simulink model "SingleJoint_Algorithm2"  (R2018b)
settings: Solver=FixedStepDiscrete  StartTime=0.0  StopTime=Inf  FixedStep=0.001  RelTol=1e-3  EnableMultiTasking=on
undefined symbols (not defined in the file): DiscIntNeverNeededParam, J3, J7, Motor_Current, Motor_Position, Motor_Velocity, Send_GUIdata
libraries: c280xlib x14, simulink x7, dspsrcs4 x1, idelinklib_common x1
(part 2 of 2)

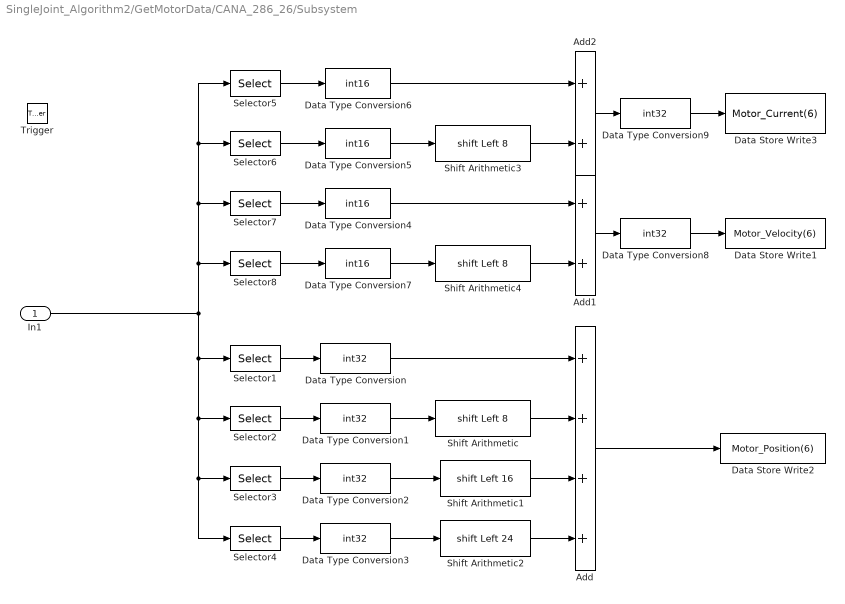
== system SingleJoint_Algorithm2/GetMotorData/CANA_286_26/Subsystem ==
  In1 : Inport
  Trigger : TriggerPort  TriggerType=function-call  VariantControl=Variant  PortDimensions=1
  Add : Sum  Inputs=4
  Add1 : Sum  Inputs=2
  Add2 : Sum  Inputs=2
  Data Store Write1 : DataStoreWrite  DataStoreName=Motor_Velocity  DataStoreElements=Motor_Velocity(6)
  Data Store Write2 : DataStoreWrite  DataStoreName=Motor_Position  DataStoreElements=Motor_Position(6)
  Data Store Write3 : DataStoreWrite  DataStoreName=Motor_Current  DataStoreElements=Motor_Current(6)
  Data Type Conversion{,1..3,8..9} (6 alike) : DataTypeConversion  OutDataTypeStr=int32
  Data Type Conversion{4..7} (4 alike) : DataTypeConversion  OutDataTypeStr=int16
  Selector1 : Selector  IndexMode=Zero-based  InputPortWidth=8  IndexOptions=Index vector (dialog)  Indices=4  OutputSizes=1
  Selector2 : Selector  IndexMode=Zero-based  InputPortWidth=8  IndexOptions=Index vector (dialog)  Indices=5  OutputSizes=1
  Selector3 : Selector  IndexMode=Zero-based  InputPortWidth=8  IndexOptions=Index vector (dialog)  Indices=6  OutputSizes=1
  Selector4 : Selector  IndexMode=Zero-based  InputPortWidth=8  IndexOptions=Index vector (dialog)  Indices=7  OutputSizes=1
  Selector5 : Selector  IndexMode=Zero-based  InputPortWidth=8  IndexOptions=Index vector (dialog)  Indices=0  OutputSizes=1
  Selector6 : Selector  IndexMode=Zero-based  InputPortWidth=8  IndexOptions=Index vector (dialog)  Indices=1  OutputSizes=1
  Selector7 : Selector  IndexMode=Zero-based  InputPortWidth=8  IndexOptions=Index vector (dialog)  Indices=2  OutputSizes=1
  Selector8 : Selector  IndexMode=Zero-based  InputPortWidth=8  IndexOptions=Index vector (dialog)  Indices=3  OutputSizes=1
  Shift Arithmetic : ArithShift  BitShiftNumber=8  BitShiftDirection=Left
  Shift Arithmetic1 : ArithShift  BitShiftNumber=16  BitShiftDirection=Left
  Shift Arithmetic2 : ArithShift  BitShiftNumber=24  BitShiftDirection=Left
  Shift Arithmetic3 : ArithShift  BitShiftNumber=8  BitShiftDirection=Left
  Shift Arithmetic4 : ArithShift  BitShiftNumber=8  BitShiftDirection=Left
  wires:
  Selector3/1 -> Data Type Conversion2/1
  Shift Arithmetic/1 -> Add/2
  Shift Arithmetic2/1 -> Add/4
  Data Type Conversion/1 -> Add/1
  Selector1/1 -> Data Type Conversion/1
  Selector4/1 -> Data Type Conversion3/1
  Add/1 -> Data Store Write2/1
  Shift Arithmetic1/1 -> Add/3
  Selector2/1 -> Data Type Conversion1/1
  Selector5/1 -> Data Type Conversion6/1
  Data Type Conversion7/1 -> Shift Arithmetic4/1
  Selector7/1 -> Data Type Conversion4/1
  Selector8/1 -> Data Type Conversion7/1
  Selector6/1 -> Data Type Conversion5/1
  In1/1 -> Selector3/1, Selector4/1, Selector2/1, Selector1/1, Selector5/1, Selector6/1, Selector7/1, Selector8/1
  Add1/1 -> Data Type Conversion8/1
  Data Type Conversion1/1 -> Shift Arithmetic/1
  Data Type Conversion2/1 -> Shift Arithmetic1/1
  Data Type Conversion3/1 -> Shift Arithmetic2/1
  Shift Arithmetic4/1 -> Add1/2
  Data Type Conversion4/1 -> Add1/1
  Data Type Conversion5/1 -> Shift Arithmetic3/1
  Data Type Conversion6/1 -> Add2/1
  Shift Arithmetic3/1 -> Add2/2
  Add2/1 -> Data Type Conversion9/1
  Data Type Conversion8/1 -> Data Store Write1/1
  Data Type Conversion9/1 -> Data Store Write3/1

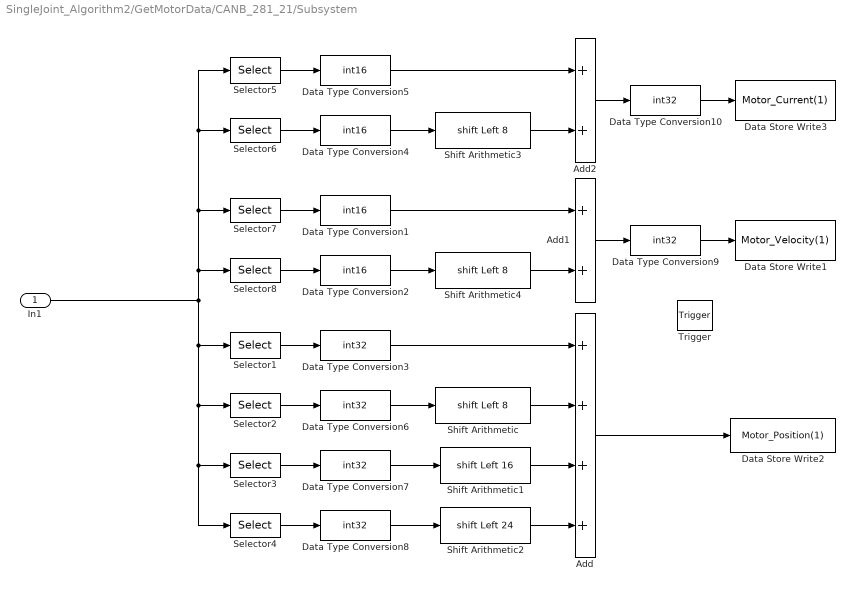
== system SingleJoint_Algorithm2/GetMotorData/CANB_281_21/Subsystem ==
  In1 : Inport
  Trigger : TriggerPort  TriggerType=function-call  VariantControl=Variant  PortDimensions=1
  Add : Sum  Inputs=4
  Add1 : Sum  Inputs=2
  Add2 : Sum  Inputs=2
  Data Store Write1 : DataStoreWrite  DataStoreName=Motor_Velocity  DataStoreElements=Motor_Velocity(1)
  Data Store Write2 : DataStoreWrite  DataStoreName=Motor_Position  DataStoreElements=Motor_Position(1)
  Data Store Write3 : DataStoreWrite  DataStoreName=Motor_Current  DataStoreElements=Motor_Current(1)
  Data Type Conversion{1..2,4..5} (4 alike) : DataTypeConversion  OutDataTypeStr=int16
  Data Type Conversion{3,6..10} (6 alike) : DataTypeConversion  OutDataTypeStr=int32
  Selector1 : Selector  IndexMode=Zero-based  InputPortWidth=8  IndexOptions=Index vector (dialog)  Indices=4  OutputSizes=1
  Selector2 : Selector  IndexMode=Zero-based  InputPortWidth=8  IndexOptions=Index vector (dialog)  Indices=5  OutputSizes=1
  Selector3 : Selector  IndexMode=Zero-based  InputPortWidth=8  IndexOptions=Index vector (dialog)  Indices=6  OutputSizes=1
  Selector4 : Selector  IndexMode=Zero-based  InputPortWidth=8  IndexOptions=Index vector (dialog)  Indices=7  OutputSizes=1
  Selector5 : Selector  IndexMode=Zero-based  InputPortWidth=8  IndexOptions=Index vector (dialog)  Indices=0  OutputSizes=1
  Selector6 : Selector  IndexMode=Zero-based  InputPortWidth=8  IndexOptions=Index vector (dialog)  Indices=1  OutputSizes=1
  Selector7 : Selector  IndexMode=Zero-based  InputPortWidth=8  IndexOptions=Index vector (dialog)  Indices=2  OutputSizes=1
  Selector8 : Selector  IndexMode=Zero-based  InputPortWidth=8  IndexOptions=Index vector (dialog)  Indices=3  OutputSizes=1
  Shift Arithmetic : ArithShift  BitShiftNumber=8  BitShiftDirection=Left
  Shift Arithmetic1 : ArithShift  BitShiftNumber=16  BitShiftDirection=Left
  Shift Arithmetic2 : ArithShift  BitShiftNumber=24  BitShiftDirection=Left
  Shift Arithmetic3 : ArithShift  BitShiftNumber=8  BitShiftDirection=Left
  Shift Arithmetic4 : ArithShift  BitShiftNumber=8  BitShiftDirection=Left
  wires:
  Data Type Conversion7/1 -> Shift Arithmetic1/1
  Shift Arithmetic/1 -> Add/2
  Selector2/1 -> Data Type Conversion6/1
  Selector3/1 -> Data Type Conversion7/1
  Shift Arithmetic2/1 -> Add/4
  Data Type Conversion3/1 -> Add/1
  Selector1/1 -> Data Type Conversion3/1
  Data Type Conversion8/1 -> Shift Arithmetic2/1
  Add/1 -> Data Store Write2/1
  Selector4/1 -> Data Type Conversion8/1
  Shift Arithmetic1/1 -> Add/3
  Data Type Conversion6/1 -> Shift Arithmetic/1
  Data Type Conversion2/1 -> Shift Arithmetic4/1
  Shift Arithmetic4/1 -> Add1/2
  Data Type Conversion1/1 -> Add1/1
  Selector7/1 -> Data Type Conversion1/1
  Selector8/1 -> Data Type Conversion2/1
  Selector6/1 -> Data Type Conversion4/1
  In1/1 -> Selector3/1, Selector4/1, Selector2/1, Selector1/1, Selector5/1, Selector6/1, Selector7/1, Selector8/1
  Add1/1 -> Data Type Conversion9/1
  Selector5/1 -> Data Type Conversion5/1
  Data Type Conversion4/1 -> Shift Arithmetic3/1
  Data Type Conversion9/1 -> Data Store Write1/1
  Shift Arithmetic3/1 -> Add2/2
  Data Type Conversion5/1 -> Add2/1
  Add2/1 -> Data Type Conversion10/1
  Data Type Conversion10/1 -> Data Store Write3/1

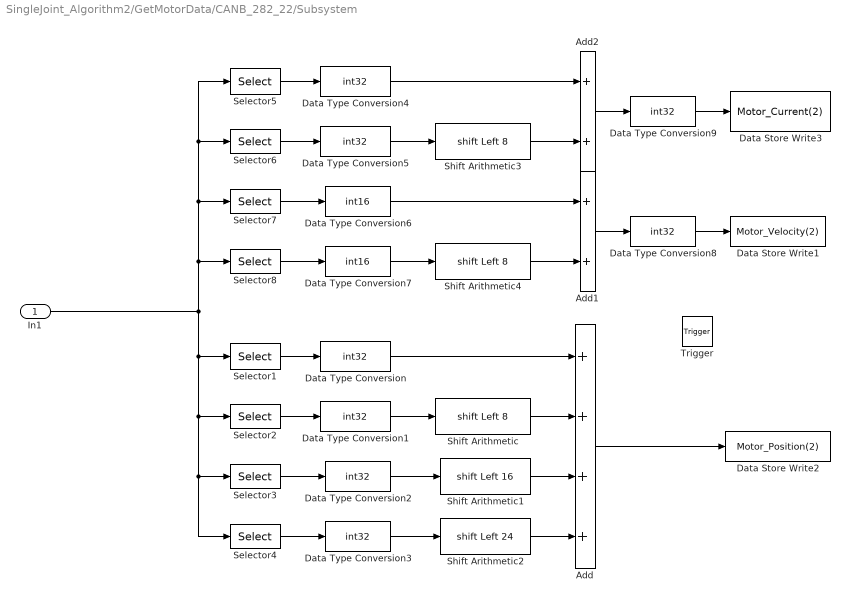
== system SingleJoint_Algorithm2/GetMotorData/CANB_282_22/Subsystem ==
  In1 : Inport
  Trigger : TriggerPort  TriggerType=function-call  VariantControl=Variant  PortDimensions=1
  Add : Sum  Inputs=4
  Add1 : Sum  Inputs=2
  Add2 : Sum  Inputs=2
  Data Store Write1 : DataStoreWrite  DataStoreName=Motor_Velocity  DataStoreElements=Motor_Velocity(2)
  Data Store Write2 : DataStoreWrite  DataStoreName=Motor_Position  DataStoreElements=Motor_Position(2)
  Data Store Write3 : DataStoreWrite  DataStoreName=Motor_Current  DataStoreElements=Motor_Current(2)
  Data Type Conversion{,1..5,8..9} (8 alike) : DataTypeConversion  OutDataTypeStr=int32
  Data Type Conversion6 : DataTypeConversion  OutDataTypeStr=int16
  Data Type Conversion7 : DataTypeConversion  OutDataTypeStr=int16
  Selector1 : Selector  IndexMode=Zero-based  InputPortWidth=8  IndexOptions=Index vector (dialog)  Indices=4  OutputSizes=1
  Selector2 : Selector  IndexMode=Zero-based  InputPortWidth=8  IndexOptions=Index vector (dialog)  Indices=5  OutputSizes=1
  Selector3 : Selector  IndexMode=Zero-based  InputPortWidth=8  IndexOptions=Index vector (dialog)  Indices=6  OutputSizes=1
  Selector4 : Selector  IndexMode=Zero-based  InputPortWidth=8  IndexOptions=Index vector (dialog)  Indices=7  OutputSizes=1
  Selector5 : Selector  IndexMode=Zero-based  InputPortWidth=8  IndexOptions=Index vector (dialog)  Indices=0  OutputSizes=1
  Selector6 : Selector  IndexMode=Zero-based  InputPortWidth=8  IndexOptions=Index vector (dialog)  Indices=1  OutputSizes=1
  Selector7 : Selector  IndexMode=Zero-based  InputPortWidth=8  IndexOptions=Index vector (dialog)  Indices=2  OutputSizes=1
  Selector8 : Selector  IndexMode=Zero-based  InputPortWidth=8  IndexOptions=Index vector (dialog)  Indices=3  OutputSizes=1
  Shift Arithmetic : ArithShift  BitShiftNumber=8  BitShiftDirection=Left
  Shift Arithmetic1 : ArithShift  BitShiftNumber=16  BitShiftDirection=Left
  Shift Arithmetic2 : ArithShift  BitShiftNumber=24  BitShiftDirection=Left
  Shift Arithmetic3 : ArithShift  BitShiftNumber=8  BitShiftDirection=Left
  Shift Arithmetic4 : ArithShift  BitShiftNumber=8  BitShiftDirection=Left
  wires:
  Data Type Conversion2/1 -> Shift Arithmetic1/1
  Shift Arithmetic/1 -> Add/2
  Selector2/1 -> Data Type Conversion1/1
  Selector3/1 -> Data Type Conversion2/1
  Shift Arithmetic2/1 -> Add/4
  Data Type Conversion/1 -> Add/1
  Selector1/1 -> Data Type Conversion/1
  Data Type Conversion3/1 -> Shift Arithmetic2/1
  Add/1 -> Data Store Write2/1
  Selector4/1 -> Data Type Conversion3/1
  Shift Arithmetic1/1 -> Add/3
  Data Type Conversion1/1 -> Shift Arithmetic/1
  In1/1 -> Selector3/1, Selector4/1, Selector2/1, Selector1/1, Selector8/1, Selector7/1, Selector6/1, Selector5/1
  Shift Arithmetic4/1 -> Add1/2
  Add1/1 -> Data Type Conversion8/1
  Data Type Conversion5/1 -> Shift Arithmetic3/1
  Selector8/1 -> Data Type Conversion7/1
  Data Type Conversion6/1 -> Add1/1
  Selector6/1 -> Data Type Conversion5/1
  Data Type Conversion7/1 -> Shift Arithmetic4/1
  Selector5/1 -> Data Type Conversion4/1
  Selector7/1 -> Data Type Conversion6/1
  Data Type Conversion8/1 -> Data Store Write1/1
  Shift Arithmetic3/1 -> Add2/2
  Data Type Conversion4/1 -> Add2/1
  Add2/1 -> Data Type Conversion9/1
  Data Type Conversion9/1 -> Data Store Write3/1

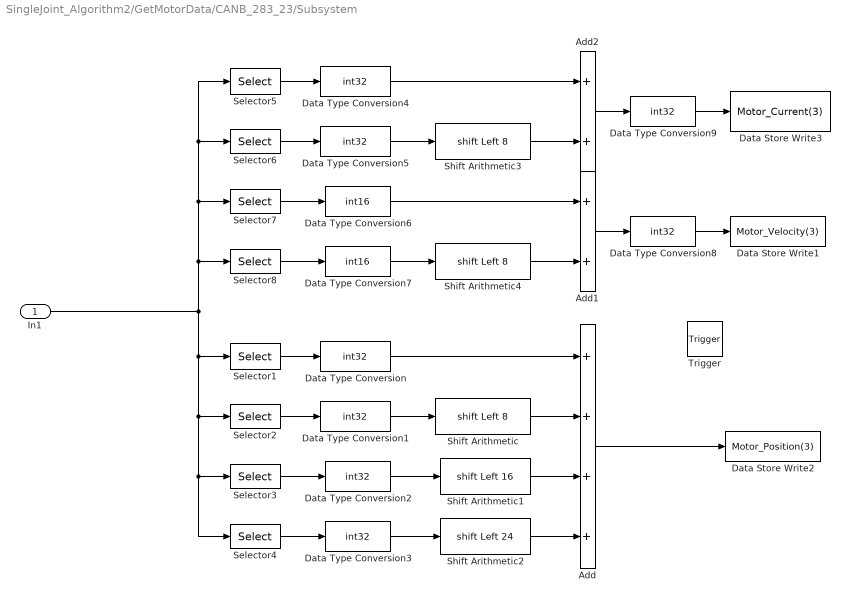
== system SingleJoint_Algorithm2/GetMotorData/CANB_283_23/Subsystem ==
  In1 : Inport
  Trigger : TriggerPort  TriggerType=function-call  VariantControl=Variant  PortDimensions=1
  Add : Sum  Inputs=4
  Add1 : Sum  Inputs=2
  Add2 : Sum  Inputs=2
  Data Store Write1 : DataStoreWrite  DataStoreName=Motor_Velocity  DataStoreElements=Motor_Velocity(3)
  Data Store Write2 : DataStoreWrite  DataStoreName=Motor_Position  DataStoreElements=Motor_Position(3)
  Data Store Write3 : DataStoreWrite  DataStoreName=Motor_Current  DataStoreElements=Motor_Current(3)
  Data Type Conversion{,1..5,8..9} (8 alike) : DataTypeConversion  OutDataTypeStr=int32
  Data Type Conversion6 : DataTypeConversion  OutDataTypeStr=int16
  Data Type Conversion7 : DataTypeConversion  OutDataTypeStr=int16
  Selector1 : Selector  IndexMode=Zero-based  InputPortWidth=8  IndexOptions=Index vector (dialog)  Indices=4  OutputSizes=1
  Selector2 : Selector  IndexMode=Zero-based  InputPortWidth=8  IndexOptions=Index vector (dialog)  Indices=5  OutputSizes=1
  Selector3 : Selector  IndexMode=Zero-based  InputPortWidth=8  IndexOptions=Index vector (dialog)  Indices=6  OutputSizes=1
  Selector4 : Selector  IndexMode=Zero-based  InputPortWidth=8  IndexOptions=Index vector (dialog)  Indices=7  OutputSizes=1
  Selector5 : Selector  IndexMode=Zero-based  InputPortWidth=8  IndexOptions=Index vector (dialog)  Indices=0  OutputSizes=1
  Selector6 : Selector  IndexMode=Zero-based  InputPortWidth=8  IndexOptions=Index vector (dialog)  Indices=1  OutputSizes=1
  Selector7 : Selector  IndexMode=Zero-based  InputPortWidth=8  IndexOptions=Index vector (dialog)  Indices=2  OutputSizes=1
  Selector8 : Selector  IndexMode=Zero-based  InputPortWidth=8  IndexOptions=Index vector (dialog)  Indices=3  OutputSizes=1
  Shift Arithmetic : ArithShift  BitShiftNumber=8  BitShiftDirection=Left
  Shift Arithmetic1 : ArithShift  BitShiftNumber=16  BitShiftDirection=Left
  Shift Arithmetic2 : ArithShift  BitShiftNumber=24  BitShiftDirection=Left
  Shift Arithmetic3 : ArithShift  BitShiftNumber=8  BitShiftDirection=Left
  Shift Arithmetic4 : ArithShift  BitShiftNumber=8  BitShiftDirection=Left
  wires:
  Data Type Conversion2/1 -> Shift Arithmetic1/1
  Shift Arithmetic/1 -> Add/2
  Selector2/1 -> Data Type Conversion1/1
  Selector3/1 -> Data Type Conversion2/1
  Shift Arithmetic2/1 -> Add/4
  Data Type Conversion/1 -> Add/1
  Selector1/1 -> Data Type Conversion/1
  Data Type Conversion3/1 -> Shift Arithmetic2/1
  Add/1 -> Data Store Write2/1
  Selector4/1 -> Data Type Conversion3/1
  Shift Arithmetic1/1 -> Add/3
  Data Type Conversion1/1 -> Shift Arithmetic/1
  Selector6/1 -> Data Type Conversion5/1
  Selector5/1 -> Data Type Conversion4/1
  Data Type Conversion7/1 -> Shift Arithmetic4/1
  Data Type Conversion6/1 -> Add1/1
  Selector7/1 -> Data Type Conversion6/1
  Selector8/1 -> Data Type Conversion7/1
  Data Type Conversion5/1 -> Shift Arithmetic3/1
  In1/1 -> Selector3/1, Selector4/1, Selector2/1, Selector1/1, Selector5/1, Selector6/1, Selector7/1, Selector8/1
  Add1/1 -> Data Type Conversion8/1
  Shift Arithmetic4/1 -> Add1/2
  Data Type Conversion8/1 -> Data Store Write1/1
  Shift Arithmetic3/1 -> Add2/2
  Data Type Conversion4/1 -> Add2/1
  Add2/1 -> Data Type Conversion9/1
  Data Type Conversion9/1 -> Data Store Write3/1

== system SingleJoint_Algorithm2/接收上位机的数据/Subsystem/Joint1 ==
  Joint1 : Inport
  Action Port : ActionPort  ActionType=case
  Data Store Write2 : DataStoreWrite  DataStoreName=J1
  wires:
  Joint1/1 -> Data Store Write2/1

== system SingleJoint_Algorithm2/接收上位机的数据/Subsystem/Joint2 ==
  Joint2 : Inport
  Action Port : ActionPort  ActionType=case
  Data Store Write2 : DataStoreWrite  DataStoreName=J2
  wires:
  Joint2/1 -> Data Store Write2/1

== system SingleJoint_Algorithm2/接收上位机的数据/Subsystem/Joint3 ==
  Joint3 : Inport
  Action Port : ActionPort  ActionType=case
  Data Store Write2 : DataStoreWrite  DataStoreName=J3
  wires:
  Joint3/1 -> Data Store Write2/1

== system SingleJoint_Algorithm2/接收上位机的数据/Subsystem/Joint4 ==
  Joint4 : Inport
  Action Port : ActionPort  ActionType=case
  Data Store Write2 : DataStoreWrite  DataStoreName=J4
  wires:
  Joint4/1 -> Data Store Write2/1

== system SingleJoint_Algorithm2/接收上位机的数据/Subsystem/Joint5 ==
  Joint5 : Inport
  Action Port : ActionPort  ActionType=case
  Data Store Write2 : DataStoreWrite  DataStoreName=J5
  wires:
  Joint5/1 -> Data Store Write2/1

== system SingleJoint_Algorithm2/接收上位机的数据/Subsystem/Joint6 ==
  Joint6 : Inport
  Action Port : ActionPort  ActionType=case
  Data Store Write2 : DataStoreWrite  DataStoreName=J6
  wires:
  Joint6/1 -> Data Store Write2/1

== system SingleJoint_Algorithm2/接收上位机的数据/Subsystem/Joint7 ==
  Joint7 : Inport
  Action Port : ActionPort  ActionType=case
  Data Store Write2 : DataStoreWrite  DataStoreName=J7
  wires:
  Joint7/1 -> Data Store Write2/1

== system SingleJoint_Algorithm2/接收上位机的数据/获取用户命令/消息校验 ==
  数据 : Inport
  Add : Sum  Inputs=8
  Constant : Constant  Value=[0 0 0 0 0 0 0 0 0]  OutDataTypeStr=uint16
  Data Type Conversion : DataTypeConversion  OutDataTypeStr=uint16
  Demux : Demux  Outputs=9
  Relational Operator : RelationalOperator  Operator===  OutDataTypeStr=boolean  RndMeth=Simplest
  Switch : Switch  Criteria=u2 > Threshold
  消息 : Outport
  使能 : Outport  Port=2
  wires:
  数据/1 -> Switch/1, Demux/1
  Demux/1 -> Add/1
  Demux/2 -> Add/2
  Demux/3 -> Add/3
  Demux/4 -> Add/4
  Demux/5 -> Add/5
  Demux/6 -> Add/6
  Demux/7 -> Add/7
  Demux/8 -> Add/8
  Add/1 -> Data Type Conversion/1
  Data Type Conversion/1 -> Relational Operator/1
  Demux/9 -> Relational Operator/2
  Switch/1 -> 消息/1
  Constant/1 -> Switch/3
  Relational Operator/1 -> Switch/2, 使能/1

== system SingleJoint_Algorithm2/AdaptionController/AdapitionController/Controller/SolveTau ==
  note: $\dot\hat\omega=-\lambda f^Ts$
  note: $f\hat\omega$
  note: $K_Ds$
  note: $\Gamma_0\eta_1$
  Gamma0 eta1 : Inport
  f : Inport  Port=2
  lambda : Inport  Port=3
  KD : Inport  Port=4
  s : Inport  Port=5
  6 : Gain  Gain=-1  OutDataTypeStr=double
  Add : Sum  Inputs=++-
  Discrete-Time Integrator2 : DiscreteIntegrator  SampleTime=-1  LimitOutput=on  UpperSaturationLimit=[1000;1000;1000;1000;1000;1000;1000;]  LowerSaturationLimit=[-1000;-1000;-1000;-1000;-1000;-1000;-1000;]  ICPrevOutput=DiscIntNeverNeededParam  ICPrevScaledInput=DiscIntNeverNeededParam
  Math Function2 : Math  Operator=transpose  SaturateOnIntegerOverflow=on
  Product5 : Product
  Product6 : Product  Inputs=3
  Product7 : Product  Multiplication=Matrix(*)
  transpose : Reshape  OutputDimensionality=Customize  OutputDimensions=[1,7]
  Tau : Outport
  wires:
  f/1 -> Math Function2/1, transpose/1
  Product6/1 -> Discrete-Time Integrator2/1
  Product7/1 -> Add/2
  Product5/1 -> Add/3
  lambda/1 -> 6/1
  Math Function2/1 -> Product6/1
  Discrete-Time Integrator2/1 -> Product7/2
  6/1 -> Product6/2
  s/1 -> Product6/3, Product5/1
  transpose/1 -> Product7/1
  KD/1 -> Product5/2
  Gamma0 eta1/1 -> Add/1
  Add/1 -> Tau/1

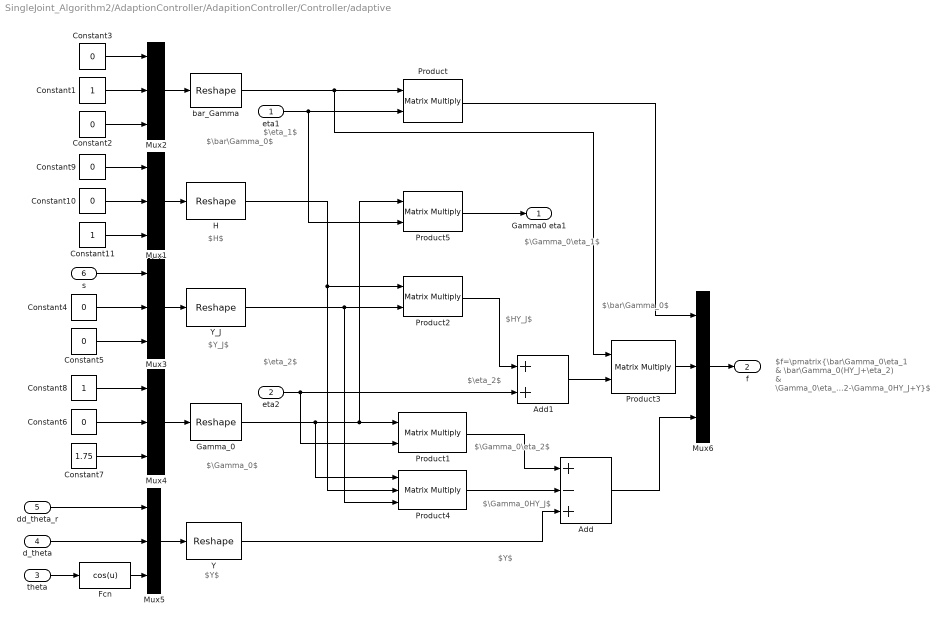
== system SingleJoint_Algorithm2/AdaptionController/AdapitionController/Controller/adaptive ==
  note: $\eta_2$
  note: $\bar\Gamma_0$
  note: $\Gamma_0$
  note: $\eta_1$
  note: $\Gamma_0\eta_1$
  note: $H$
  note: $Y_J$
  note: $Y$
  note: $HY_J$
  note: $\Gamma_0\eta_2$
  note: $\Gamma_0HY_J$
  note: $Y$
  note: $\eta_2$
  note: $\bar\Gamma_0$
  note: $f=\pmatrix{\bar\Gamma_0\eta_1 & \bar\Gamma_0(HY_J+\eta_2) & \Gamma_0\eta_2-\Gamma_0HY_J+Y}$
  eta1 : Inport
  eta2 : Inport  Port=2
  theta : Inport  Port=3
  d_theta : Inport  Port=4
  dd_theta_r : Inport  Port=5
  s : Inport  Port=6
  Add : Sum  Inputs=+-+
  Add1 : Sum
  Constant1 : Constant
  Constant{2..6,9..10} (7 alike) : Constant  Value=0
  Constant11 : Constant
  Constant7 : Constant  Value=1.75
  Constant8 : Constant
  Fcn : Fcn  Expr=cos(u)
  Gamma_0 : Reshape  OutputDimensionality=Customize  OutputDimensions=[1,3]
  H : Reshape  OutputDimensionality=Customize  OutputDimensions=[3,1]
  Mux{1..6} (6 alike) : Mux  Inputs=3
  Product{,1..3,5} (5 alike) : Product  Multiplication=Matrix(*)
  Product4 : Product  Inputs=3  Multiplication=Matrix(*)
  Y : Reshape  OutputDimensionality=Customize  OutputDimensions=[1,3]
  Y_J : Reshape  OutputDimensionality=Customize  OutputDimensions=[1,3]
  bar_Gamma : Reshape  OutputDimensionality=Customize  OutputDimensions=[1,3]
  Gamma0 eta1 : Outport
  f : Outport  Port=2
  wires:
  H/1 -> Product4/2, Product2/1
  Mux1/1 -> H/1
  Constant11/1 -> Mux1/3
  Constant10/1 -> Mux1/2
  Constant9/1 -> Mux1/1
  bar_Gamma/1 -> Product/1, Product3/1
  Constant2/1 -> Mux2/3
  Constant1/1 -> Mux2/2
  Constant3/1 -> Mux2/1
  Mux2/1 -> bar_Gamma/1
  eta1/1 -> Product5/2, Product/2
  Mux3/1 -> Y_J/1
  Constant5/1 -> Mux3/3
  Constant4/1 -> Mux3/2
  s/1 -> Mux3/1
  Y_J/1 -> Product2/2, Product4/3
  Product2/1 -> Add1/1
  eta2/1 -> Product1/2, Add1/2
  Add1/1 -> Product3/2
  Mux4/1 -> Gamma_0/1
  Constant7/1 -> Mux4/3
  Constant6/1 -> Mux4/2
  Constant8/1 -> Mux4/1
  Gamma_0/1 -> Product4/1, Product5/1, Product1/1
  dd_theta_r/1 -> Mux5/1
  d_theta/1 -> Mux5/2
  theta/1 -> Fcn/1
  Fcn/1 -> Mux5/3
  Mux5/1 -> Y/1
  Y/1 -> Add/3
  Product4/1 -> Add/2
  Product1/1 -> Add/1
  Product3/1 -> Mux6/2
  Product/1 -> Mux6/1
  Mux6/1 -> f/1
  Add/1 -> Mux6/3
  Product5/1 -> Gamma0 eta1/1

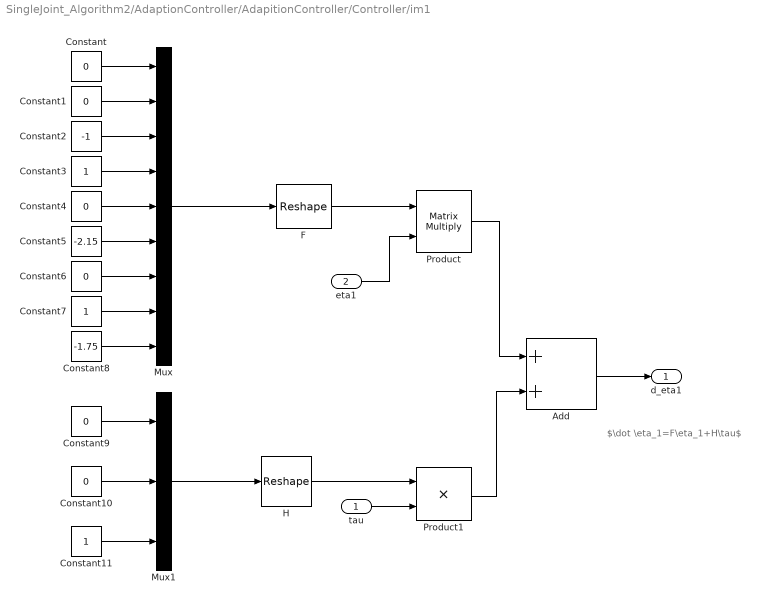
== system SingleJoint_Algorithm2/AdaptionController/AdapitionController/Controller/im1 ==
  note: $\dot \eta_1=F\eta_1+H\tau$
  tau : Inport
  eta1 : Inport  Port=2
  Add : Sum
  Constant{,1,4,6,9..10} (6 alike) : Constant  Value=0
  Constant11 : Constant
  Constant2 : Constant  Value=-1
  Constant3 : Constant
  Constant5 : Constant  Value=-2.15
  Constant7 : Constant
  Constant8 : Constant  Value=-1.75
  F : Reshape  OutputDimensionality=Customize  OutputDimensions=[3,3]
  H : Reshape  OutputDimensionality=Customize  OutputDimensions=[3,1]
  Mux : Mux  Inputs=9
  Mux1 : Mux  Inputs=3
  Product : Product  Multiplication=Matrix(*)
  Product1 : Product
  d_eta1 : Outport
  wires:
  Constant/1 -> Mux/1
  Constant1/1 -> Mux/2
  Constant2/1 -> Mux/3
  Constant3/1 -> Mux/4
  Constant4/1 -> Mux/5
  Constant5/1 -> Mux/6
  Constant6/1 -> Mux/7
  Constant7/1 -> Mux/8
  Constant8/1 -> Mux/9
  Mux/1 -> F/1
  F/1 -> Product/1
  Product/1 -> Add/1
  Constant9/1 -> Mux1/1
  Constant10/1 -> Mux1/2
  Constant11/1 -> Mux1/3
  Mux1/1 -> H/1
  H/1 -> Product1/1
  tau/1 -> Product1/2
  Product1/1 -> Add/2
  Add/1 -> d_eta1/1
  eta1/1 -> Product/2

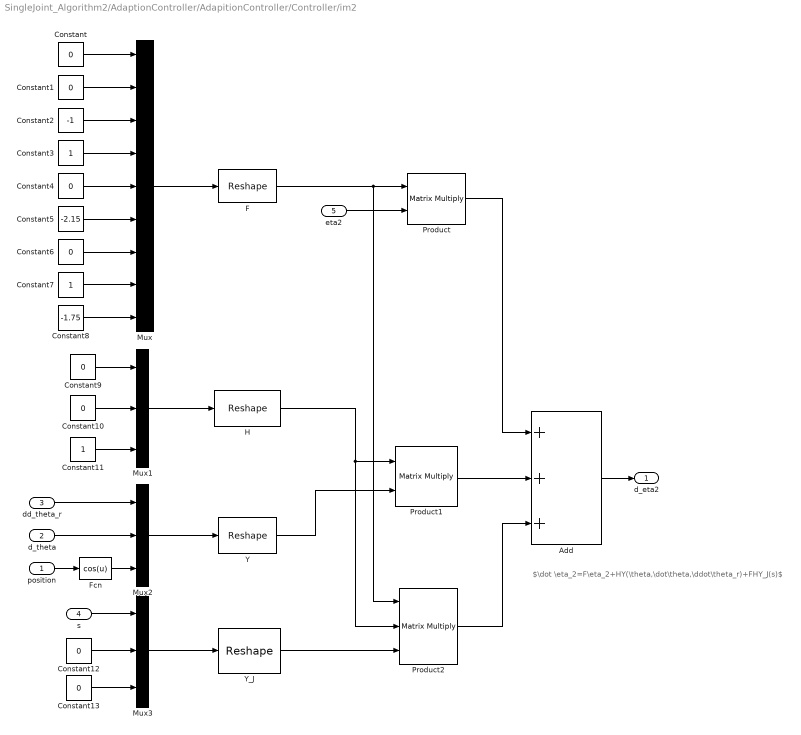
== system SingleJoint_Algorithm2/AdaptionController/AdapitionController/Controller/im2 ==
  note: $\dot \eta_2=F\eta_2+HY(\theta,\dot\theta,\ddot\theta_r)+FHY_J(s)$
  position : Inport
  d_theta : Inport  Port=2
  dd_theta_r : Inport  Port=3
  s : Inport  Port=4
  eta2 : Inport  Port=5
  Add : Sum  Inputs=+++
  Constant{,1,4,6,9..10,12..13} (8 alike) : Constant  Value=0
  Constant11 : Constant
  Constant2 : Constant  Value=-1
  Constant3 : Constant
  Constant5 : Constant  Value=-2.15
  Constant7 : Constant
  Constant8 : Constant  Value=-1.75
  F : Reshape  OutputDimensionality=Customize  OutputDimensions=[3,3]
  Fcn : Fcn  Expr=cos(u)
  H : Reshape  OutputDimensionality=Customize  OutputDimensions=[3,1]
  Mux : Mux  Inputs=9
  Mux1 : Mux  Inputs=3
  Mux2 : Mux  Inputs=3
  Mux3 : Mux  Inputs=3
  Product : Product  Multiplication=Matrix(*)
  Product1 : Product  Multiplication=Matrix(*)
  Product2 : Product  Inputs=3  Multiplication=Matrix(*)
  Y : Reshape  OutputDimensionality=Customize  OutputDimensions=[1,3]
  Y_J : Reshape  OutputDimensionality=Customize  OutputDimensions=[1,3]
  d_eta2 : Outport
  wires:
  eta2/1 -> Product/2
  Add/1 -> d_eta2/1
  Product1/1 -> Add/2
  H/1 -> Product2/2, Product1/1
  Mux1/1 -> H/1
  Constant11/1 -> Mux1/3
  Constant10/1 -> Mux1/2
  Constant9/1 -> Mux1/1
  Product/1 -> Add/1
  F/1 -> Product2/1, Product/1
  Mux/1 -> F/1
  Constant8/1 -> Mux/9
  Constant7/1 -> Mux/8
  Constant6/1 -> Mux/7
  Constant5/1 -> Mux/6
  Constant4/1 -> Mux/5
  Constant3/1 -> Mux/4
  Constant2/1 -> Mux/3
  Constant1/1 -> Mux/2
  Constant/1 -> Mux/1
  dd_theta_r/1 -> Mux2/1
  d_theta/1 -> Mux2/2
  position/1 -> Fcn/1
  Fcn/1 -> Mux2/3
  Mux2/1 -> Y/1
  Y/1 -> Product1/2
  s/1 -> Mux3/1
  Constant12/1 -> Mux3/2
  Constant13/1 -> Mux3/3
  Mux3/1 -> Y_J/1
  Y_J/1 -> Product2/3
  Product2/1 -> Add/3

== system SingleJoint_Algorithm2/AdaptionController/AdapitionController/Error/Subsystem ==
  note: $e_1(t)=\theta(t)-\theta_d(t)$
  q1 : Inport
  gian : Inport  Port=2
  Enable : EnablePort
  Product : Product
  Sum5 : Sum  Inputs=+-|
  ref_signal : dspsrcs4/Sine Wave  Amplitude=1  Frequency=Freq  Phase=0  SampleMode=Discrete  OutComplex=Real  CompMethod=Trigonometric fcn  TableSize=Speed  SampleTime=SimpleTime  SamplesPerFrame=1  ResetState=Restart at time zero  OutputFrames=on  dataType=double  wordLen=16  udDataType=sfix(16)  fracBitsMode=Best precision  numFracBits=15  OutDataTypeStr=double  LastOutDataTypeStr=double
  e1 : Outport
  qd : Outport  Port=2
  wires:
  ref_signal/1 -> Product/1
  Product/1 -> Sum5/2, qd/1
  gian/1 -> Product/2
  q1/1 -> Sum5/1
  Sum5/1 -> e1/1

== system SingleJoint_Algorithm2/AdaptionController/DriverOneMotor/BottomDriver/Joint1 ==
  In6 : Inport
  Action Port : ActionPort
  Constant : Constant  Value=0  OutDataTypeStr=uint8
  Data Store Write : DataStoreWrite  DataStoreName=One_TXD
  eCANB_301_7 : c280xlib/eCAN Transmit  chipFamily=C280x  useModule=eCAN_B  mailboxNo=7  messageID=hex2dec('301')  messageType=Standard (11-bit identifier)  enableBlockingMode=off  postInterrupt=off  interruptLine=0
      settings: SourceProductName=Embedded Coder Support Package for Texas Instruments C2000 Processors  SourceProductBaseCode=TIC2000
  wires:
  In6/1 -> eCANB_301_7/1
  Constant/1 -> Data Store Write/1

== system SingleJoint_Algorithm2/AdaptionController/DriverOneMotor/BottomDriver/Joint2 ==
  In1 : Inport
  Action Port : ActionPort
  Constant : Constant  Value=0  OutDataTypeStr=uint8
  Data Store Write : DataStoreWrite  DataStoreName=One_TXD
  eCANB _302_7 : c280xlib/eCAN Transmit  chipFamily=C280x  useModule=eCAN_B  mailboxNo=7  messageID=hex2dec('302')  messageType=Standard (11-bit identifier)  enableBlockingMode=off  postInterrupt=off  interruptLine=0
      settings: SourceProductName=Embedded Coder Support Package for Texas Instruments C2000 Processors  SourceProductBaseCode=TIC2000
  wires:
  In1/1 -> eCANB _302_7/1
  Constant/1 -> Data Store Write/1

== system SingleJoint_Algorithm2/AdaptionController/DriverOneMotor/BottomDriver/Joint3 ==
  In1 : Inport
  Action Port : ActionPort  ActionType=case
  Constant : Constant  Value=0  OutDataTypeStr=uint8
  Data Store Write : DataStoreWrite  DataStoreName=One_TXD
  eCANB _303_7 : c280xlib/eCAN Transmit  chipFamily=C280x  useModule=eCAN_B  mailboxNo=7  messageID=hex2dec('303')  messageType=Standard (11-bit identifier)  enableBlockingMode=off  postInterrupt=off  interruptLine=0
      settings: SourceProductName=Embedded Coder Support Package for Texas Instruments C2000 Processors  SourceProductBaseCode=TIC2000
  wires:
  In1/1 -> eCANB _303_7/1
  Constant/1 -> Data Store Write/1

== system SingleJoint_Algorithm2/AdaptionController/DriverOneMotor/BottomDriver/Joint4 ==
  In1 : Inport
  Action Port : ActionPort
  Constant : Constant  Value=0  OutDataTypeStr=uint8
  Data Store Write : DataStoreWrite  DataStoreName=One_TXD
  eCANA_304_7 : c280xlib/eCAN Transmit  chipFamily=C280x  useModule=eCAN_A  mailboxNo=7  messageID=hex2dec('304')  messageType=Standard (11-bit identifier)  enableBlockingMode=off  postInterrupt=off  interruptLine=0
      settings: SourceProductName=Embedded Coder Support Package for Texas Instruments C2000 Processors  SourceProductBaseCode=TIC2000
  wires:
  In1/1 -> eCANA_304_7/1
  Constant/1 -> Data Store Write/1

== system SingleJoint_Algorithm2/AdaptionController/DriverOneMotor/BottomDriver/Joint5 ==
  In1 : Inport
  Action Port : ActionPort
  Constant : Constant  Value=0  OutDataTypeStr=uint8
  Data Store Write : DataStoreWrite  DataStoreName=One_TXD
  eCANA_305_7 : c280xlib/eCAN Transmit  chipFamily=C280x  useModule=eCAN_A  mailboxNo=7  messageID=hex2dec('305')  messageType=Standard (11-bit identifier)  enableBlockingMode=off  postInterrupt=off  interruptLine=0
      settings: SourceProductName=Embedded Coder Support Package for Texas Instruments C2000 Processors  SourceProductBaseCode=TIC2000
  wires:
  In1/1 -> eCANA_305_7/1
  Constant/1 -> Data Store Write/1

== system SingleJoint_Algorithm2/AdaptionController/DriverOneMotor/BottomDriver/Joint6 ==
  In1 : Inport
  Action Port : ActionPort
  Constant : Constant  Value=0  OutDataTypeStr=uint8
  Data Store Write : DataStoreWrite  DataStoreName=One_TXD
  eCANA_306_7 : c280xlib/eCAN Transmit  chipFamily=C280x  useModule=eCAN_A  mailboxNo=7  messageID=hex2dec('306')  messageType=Standard (11-bit identifier)  enableBlockingMode=off  postInterrupt=off  interruptLine=0
      settings: SourceProductName=Embedded Coder Support Package for Texas Instruments C2000 Processors  SourceProductBaseCode=TIC2000
  wires:
  In1/1 -> eCANA_306_7/1
  Constant/1 -> Data Store Write/1

== system SingleJoint_Algorithm2/AdaptionController/DriverOneMotor/驱动器指令/DriveOder/BG ==
  note: 命令
  note: 电流
  note: 位
      | 置
  f : TriggerPort  TriggerType=function-call  VariantControl=(inherit)
      settings: CopyFcn=Stateflow.SLINSF.SimulinkMan.removeBlockPreDeleteFcn  PreDeleteFcn=Stateflow.SLINSF.SimulinkMan.unsafePredeleteFcn
  Constant1 : Constant  Value=hex2dec('47')  OutDataTypeStr=uint8
  Constant2 : Constant  Value=0  VectorParams1D=off  OutDataTypeStr=uint8  SampleTime=-1
  Constant3 : Constant  Value=0  VectorParams1D=off  OutDataTypeStr=uint8  SampleTime=-1
  Constant6 : Constant  OutDataTypeStr=uint8
  Constant8 : Constant  Value=hex2dec('42')  OutDataTypeStr=uint8
  Data Store Write : DataStoreWrite  DataStoreName=One_TXD
  Data Type Conversion : DataTypeConversion  OutDataTypeStr=uint16
  Data Type Conversion{1..6} (6 alike) : DataTypeConversion  OutDataTypeStr=uint8
  Mux3 : Mux  Inputs=8
  Shift Arithmetic1 : ArithShift  BitShiftNumber=8  BitShiftDirection=Right
  Shift Arithmetic2 : ArithShift  BitShiftNumber=16  BitShiftDirection=Right
  Shift Arithmetic3 : ArithShift  BitShiftNumber=24  BitShiftDirection=Right
  Shift Arithmetic4 : ArithShift  BitShiftNumber=8  BitShiftDirection=Right
  MSG : Outport  OutDataTypeStr=uint16  PortDimensions=8
  wires:
  Constant6/1 -> Data Store Write/1
  Data Type Conversion2/1 -> Mux3/5
  Constant3/1 -> Data Type Conversion2/1, Shift Arithmetic1/1, Shift Arithmetic2/1, Shift Arithmetic3/1
  Data Type Conversion5/1 -> Mux3/8
  Data Type Conversion4/1 -> Mux3/7
  Constant1/1 -> Mux3/2
  Constant8/1 -> Mux3/1
  Mux3/1 -> Data Type Conversion/1
  Data Type Conversion6/1 -> Mux3/4
  Data Type Conversion3/1 -> Mux3/6
  Shift Arithmetic2/1 -> Data Type Conversion4/1
  Data Type Conversion1/1 -> Mux3/3
  Constant2/1 -> Shift Arithmetic4/1, Data Type Conversion1/1
  Shift Arithmetic3/1 -> Data Type Conversion5/1
  Shift Arithmetic4/1 -> Data Type Conversion6/1
  Shift Arithmetic1/1 -> Data Type Conversion3/1
  Data Type Conversion/1 -> MSG/1

== system SingleJoint_Algorithm2/AdaptionController/DriverOneMotor/驱动器指令/DriveOder/TF ==
  note: 命令
  note: 位
      | 置
  note: 电流
  Current : Inport  OutDataTypeStr=uint16  PortDimensions=1
  f : TriggerPort  TriggerType=function-call  VariantControl=(inherit)
      settings: CopyFcn=Stateflow.SLINSF.SimulinkMan.removeBlockPreDeleteFcn  PreDeleteFcn=Stateflow.SLINSF.SimulinkMan.unsafePredeleteFcn
  Constant1 : Constant  Value=hex2dec('46')  OutDataTypeStr=uint8
  Constant2 : Constant  OutDataTypeStr=uint8
  Constant3 : Constant  Value=0  VectorParams1D=off  OutDataTypeStr=uint8  SampleTime=-1
  Constant8 : Constant  Value=hex2dec('54')  OutDataTypeStr=uint8
  Data Store Write : DataStoreWrite  DataStoreName=One_TXD
  Data Type Conversion : DataTypeConversion  OutDataTypeStr=uint16
  Data Type Conversion{1..6} (6 alike) : DataTypeConversion  OutDataTypeStr=uint8
  Mux3 : Mux  Inputs=8
  Shift Arithmetic1 : ArithShift  BitShiftNumber=8  BitShiftDirection=Right
  Shift Arithmetic2 : ArithShift  BitShiftNumber=16  BitShiftDirection=Right
  Shift Arithmetic3 : ArithShift  BitShiftNumber=24  BitShiftDirection=Right
  Shift Arithmetic4 : ArithShift  BitShiftNumber=8  BitShiftDirection=Right
  MSG : Outport  OutDataTypeStr=uint16  PortDimensions=8
  wires:
  Shift Arithmetic2/1 -> Data Type Conversion4/1
  Data Type Conversion4/1 -> Mux3/7
  Data Type Conversion3/1 -> Mux3/6
  Shift Arithmetic1/1 -> Data Type Conversion3/1
  Constant3/1 -> Shift Arithmetic3/1, Shift Arithmetic2/1, Shift Arithmetic1/1, Data Type Conversion2/1
  Constant8/1 -> Mux3/1
  Mux3/1 -> Data Type Conversion/1
  Data Type Conversion5/1 -> Mux3/8
  Data Type Conversion6/1 -> Mux3/4
  Data Type Conversion1/1 -> Mux3/3
  Constant1/1 -> Mux3/2
  Shift Arithmetic4/1 -> Data Type Conversion6/1
  Data Type Conversion2/1 -> Mux3/5
  Shift Arithmetic3/1 -> Data Type Conversion5/1
  Current/1 -> Shift Arithmetic4/1, Data Type Conversion1/1
  Constant2/1 -> Data Store Write/1
  Data Type Conversion/1 -> MSG/1

== system SingleJoint_Algorithm2/AdaptionController/DriverOneMotor/驱动器指令/DriveOder/UM1 ==
  note: 命令
  note: 位
      | 置
  note: 电流
  f : TriggerPort  TriggerType=function-call  VariantControl=(inherit)
      settings: CopyFcn=Stateflow.SLINSF.SimulinkMan.removeBlockPreDeleteFcn  PreDeleteFcn=Stateflow.SLINSF.SimulinkMan.unsafePredeleteFcn
  Constant : Constant  OutDataTypeStr=uint8
  Constant1 : Constant  Value=hex2dec('4d')  OutDataTypeStr=uint8
  Constant2 : Constant  Value=0  VectorParams1D=off  OutDataTypeStr=uint8  SampleTime=-1
  Constant3 : Constant  VectorParams1D=off  OutDataTypeStr=uint8  SampleTime=-1
  Constant8 : Constant  Value=hex2dec('55')  OutDataTypeStr=uint8
  Data Store Write : DataStoreWrite  DataStoreName=One_TXD
  Data Type Conversion : DataTypeConversion  OutDataTypeStr=uint16
  Data Type Conversion{1..6} (6 alike) : DataTypeConversion  OutDataTypeStr=uint8
  Mux3 : Mux  Inputs=8
  Shift Arithmetic1 : ArithShift  BitShiftNumber=8  BitShiftDirection=Right
  Shift Arithmetic2 : ArithShift  BitShiftNumber=16  BitShiftDirection=Right
  Shift Arithmetic3 : ArithShift  BitShiftNumber=24  BitShiftDirection=Right
  Shift Arithmetic4 : ArithShift  BitShiftNumber=8  BitShiftDirection=Right
  MSG : Outport  OutDataTypeStr=uint16  PortDimensions=8
  wires:
  Constant8/1 -> Mux3/1
  Constant2/1 -> Data Type Conversion1/1, Shift Arithmetic4/1
  Data Type Conversion2/1 -> Mux3/5
  Constant3/1 -> Shift Arithmetic3/1, Shift Arithmetic2/1, Data Type Conversion2/1, Shift Arithmetic1/1
  Shift Arithmetic1/1 -> Data Type Conversion3/1
  Constant1/1 -> Mux3/2
  Shift Arithmetic3/1 -> Data Type Conversion5/1
  Data Type Conversion5/1 -> Mux3/8
  Data Type Conversion6/1 -> Mux3/4
  Data Type Conversion3/1 -> Mux3/6
  Shift Arithmetic4/1 -> Data Type Conversion6/1
  Data Type Conversion1/1 -> Mux3/3
  Shift Arithmetic2/1 -> Data Type Conversion4/1
  Data Type Conversion4/1 -> Mux3/7
  Mux3/1 -> Data Type Conversion/1
  Constant/1 -> Data Store Write/1
  Data Type Conversion/1 -> MSG/1

== system SingleJoint_Algorithm2/AdaptionController/DriverOneMotor/驱动器指令/DriveOder/check ==
  write : Inport  OutDataTypeStr=uint16  PortDimensions=1
  f : TriggerPort  TriggerType=function-call  VariantControl=(inherit)
      settings: CopyFcn=Stateflow.SLINSF.SimulinkMan.removeBlockPreDeleteFcn  PreDeleteFcn=Stateflow.SLINSF.SimulinkMan.unsafePredeleteFcn
  Constant : Constant  OutDataTypeStr=uint16
  Constant1 : Constant  Value=0  OutDataTypeStr=uint16
  Data Type Conversion : DataTypeConversion  OutDataTypeStr=uint16
  Switch : Switch  Criteria=u2 > Threshold  OutDataTypeStr=uint16
  bx : Outport  OutDataTypeStr=uint16  PortDimensions=1
  wires:
  Switch/1 -> Data Type Conversion/1
  Constant1/1 -> Switch/3
  Constant/1 -> Switch/1
  write/1 -> Switch/2
  Data Type Conversion/1 -> bx/1

== system SingleJoint_Algorithm2/AdaptionController/DriverOneMotor/驱动器指令/DriveOder/start_arm ==
  StartRobot : Inport  OutDataTypeStr=uint16  PortDimensions=1
  f : TriggerPort  TriggerType=function-call  VariantControl=(inherit)
      settings: CopyFcn=Stateflow.SLINSF.SimulinkMan.removeBlockPreDeleteFcn  PreDeleteFcn=Stateflow.SLINSF.SimulinkMan.unsafePredeleteFcn
  Constant : Constant  OutDataTypeStr=uint16
  StartRobotSubsystem : Subsystem
      settings: RTWSystemCode=Nonreusable function
  start : Outport  OutDataTypeStr=uint16  PortDimensions=1
  wires:
  StartRobot/1 -> StartRobotSubsystem/Enable
  StartRobotSubsystem/1(Out1) -> start/1
  Constant/1 -> StartRobotSubsystem/1(In1)

== system SingleJoint_Algorithm2/AdaptionController/DriverOneMotor/驱动器指令/DriveOder/start_arm/StartRobotSubsystem ==
  In1 : Inport
  Enable : EnablePort
  System Outputs : Subsystem  mask(System Outputs){ShowInLibBrowser=0}
      mask prompts: ShowInLibBrowser "Simulink:masks:CustCodeMaskParam1_MP"
      settings: CopyFcn=cccopyfcn(gcb)  OpenFcn=ccopenfcn('System Outputs Function')
      mask Help: eval('feval(''rtwprivate'',''rtwhelpview'',''rtw_sys_outputs_block'')');
      mask Display: disp('System\nOutputs');
  Out1 : Outport
  wires:
  In1/1 -> Out1/1

== system SingleJoint_Algorithm2/AdaptionController/DriverOneMotor/驱动器指令/DriveOder/start_arm/StartRobotSubsystem/System Outputs ==

== stateflow chart SingleJoint_Algorithm2/AdaptionController/DriverOneMotor/驱动器指令/DriveOder ==
  state State03
    entry:
    MSG=BG
    %开始执行
  state State02
    entry:
    MSG=UM1
    %切换到电流模式
  state State04
    during:
    MSG=TF(Current);
    %电流前馈
  state State01
    entry:
    start=0;
    during:
    start=start_arm(StartRobot)
    %启动机械臂
  state State05
    entry:
    bx=0;
    during:
    bx=check(write)
  state MSG = UM1 [function]
  state MSG = BG [function]
  state MSG = TF(Current) [function]
  state start = start_arm(StartRobot) [function]
  state bx = check(write) [function]
  (default) -> State01
  State02 -> State03 : after(0.5,sec)
  State03 -> State04 : after(0.5,sec)
  State05 -> State02 : [bx>0]
  State01 -> State05 : [start>0]
  data: MSG function_output uint16 size=8; MSG function_output uint16 size=8; Current function_input uint16 size=1; MSG function_output uint16 size=8; StartRobot function_input uint16 size=1; start function_output uint16 size=1; write function_input uint16 size=1; bx function_output uint16 size=1; Current input size=1; MSG output uint16 size=[8 1]; start local uint16; StartRobot input uint16; write input; bx local uint16
